simulink model "solution_ecuations"  (R2025a)
settings: Solver=VariableStepAuto  StartTime=0.0  StopTime=10.0  RelTol=1e-3
undefined symbols (not defined in the file): A, F, Ti
libraries: simulink x1
settings Model: Creator=Pablo  LastModifiedBy=Pablo

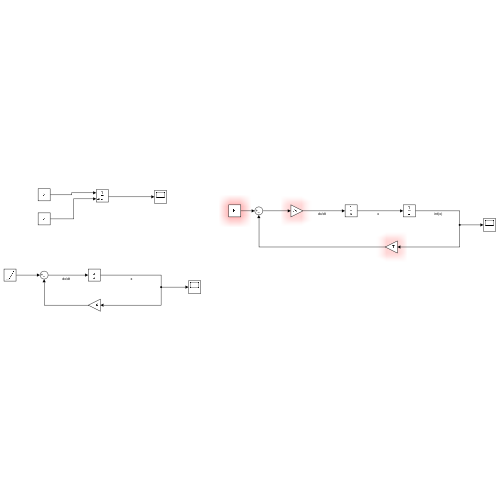
[thumbnail: Simulink's stored preview of the top-level diagram]
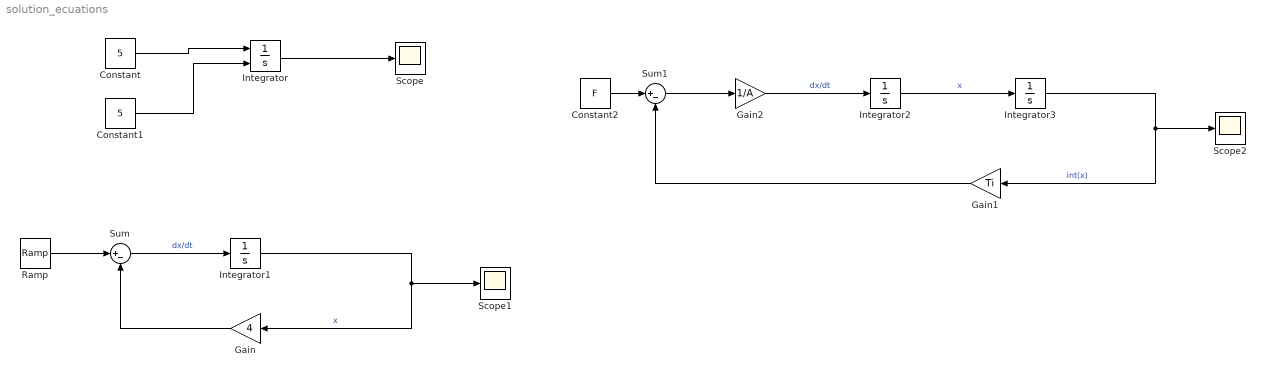
== system solution_ecuations ==
  Constant : Constant  Value=5
  Constant1 : Constant  Value=5
  Constant2 : Constant  Value=F
  Gain : Gain  Gain=4
  Gain1 : Gain  Gain=Ti
  Gain2 : Gain  Gain=1/A
  Integrator : Integrator  InitialConditionSource=external
  Integrator1 : Integrator
  Integrator2 : Integrator
  Integrator3 : Integrator
  Ramp : simulink/Sources/Ramp  slope=1  start=0  InitialOutput=0
  Scope : Scope
      settings: ActiveDisplayYMinimum=-1  ActiveDisplayYMaximum=1
  Scope1 : Scope
      settings: ActiveDisplayYMinimum=-0.3046875  ActiveDisplayYMaximum=2.7421875000000004
  Scope2 : Scope
      settings: ActiveDisplayYMinimum=-0.3046875  ActiveDisplayYMaximum=2.7421875000000004  DataLoggingVariableName=ScopeData2
  Sum : Sum  Inputs=|+-
  Sum1 : Sum  Inputs=|+-
  wires:
  Constant/1 -> Integrator/1
  Integrator/1 -> Scope/1
  Constant1/1 -> Integrator/2
  Sum/1 -> Integrator1/1  "dx/dt"
  Integrator1/1 -> Scope1/1, Gain/1  "x"
  Gain/1 -> Sum/2
  Ramp/1 -> Sum/1
  Integrator2/1 -> Integrator3/1  "x"
  Integrator3/1 -> Scope2/1, Gain1/1  "int(x)"
  Constant2/1 -> Sum1/1
  Gain1/1 -> Sum1/2
  Sum1/1 -> Gain2/1
  Gain2/1 -> Integrator2/1  "dx/dt"
